simulink model "last_test"  (Simulink 7.1)
settings: Solver=ode3  StartTime=0.0  StopTime=700.0  FixedStep=0.1  RelTol=1e-3
undefined symbols (not defined in the file or in its folder): camview, kalmanfilter4
libraries: fordypningsprosjekt x7, simulink x1
settings Model: Creator=anderga  LastModifiedBy=anders
settings OptimizationCC: SimCompilerOptimization=On

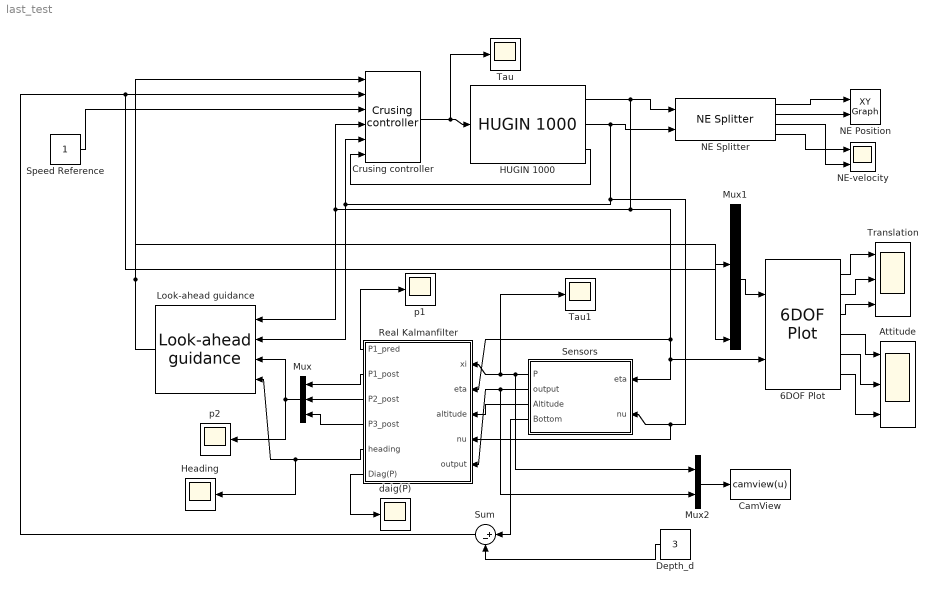
== system last_test ==
  6DOF Plot : fordypningsprosjekt/6DOF Plot  SystemSampleTime=-1
  Attitude : Scope  NumInputPorts=3
      settings: TimeRange=700  YMin=-0.5~-10~-25  YMax=0.7~1~150  SaveName=Attitude
  CamView : MATLABFcn  MATLABFcn=camview(u)
  Crusing controller : fordypningsprosjekt/Crusing controller  SystemSampleTime=-1  Kp_u=10  Ki_u=3  Kp_c=100  Kd_c=50  Kp_d=50  Kp2_d=20  Kd_d=20
  Depth_d : Constant  Orientation=left  Value=3  OutDataType=sfix(16)  OutScaling=2^0
  HUGIN 1000 : fordypningsprosjekt/HUGIN 1000  SystemSampleTime=-1  eta_0=[-30 -30 0 0 0 0]  nu_0=[0 0 0 0 0 0]  c_on_off=on  beta_c=-45  V_c=0.3
  Heading : Scope
      settings: YMin=1.3258  YMax=1.32584  SaveName=Pipeline_heading
  Look-ahead guidance : fordypningsprosjekt/Look-ahead guidance  Orientation=left  SystemSampleTime=-1
  Mux : Mux  Orientation=left  Inputs=3
  Mux1 : Mux  Inputs=6
  Mux2 : Mux  Inputs=2
  NE Position : simulink/Sinks/XY Graph  SystemSampleTime=-1  xmin=-1000  xmax=1000  ymin=-1000  ymax=1000  st=-1
  NE Splitter : fordypningsprosjekt/NE Splitter  SystemSampleTime=-1
  NE-velocity : Scope  NumInputPorts=2
      settings: YMin=1.00005~-1.87e-006  YMax=1.00011~-1.8e-006  SaveName=NE_Veloc
  Real Kalmanfilter : Subsystem  Orientation=left  AncestorBlock=fordypningsprosjekt/Real Kalmanfilter
  Sensors : Subsystem  Orientation=left  AncestorBlock=fordypningsprosjekt/Sensors
  Speed Reference : Constant  OutDataType=sfix(16)  OutScaling=2^0
  Sum : Sum  Orientation=left  Inputs=|+-  OutDataType=sfix(16)  OutScaling=2^0
  Tau : Scope
      settings: YMin=-20  YMax=110
  Tau1 : Scope
      settings: TimeRange=700  YMin=-0.5  YMax=0.5  SaveName=Cam_output
  Translation : Scope  NumInputPorts=3
      settings: YMin=-40~-50~0  YMax=30~125~10  SaveName=Translation
  daig(P) : Scope
      settings: YMin=-3.46945e-18  YMax=0.1  SaveName=diag_p_apr
  p1 : Scope
      settings: YMin=-200  YMax=600  SaveName=P_pred
  p2 : Scope
      settings: YMin=-200  YMax=600  SaveName=P_post
  wires:
  Crusing controller/1 -> HUGIN 1000/1, Tau/1
  HUGIN 1000/1 -> NE Splitter/1, Real Kalmanfilter/2(eta), Sensors/1(eta), 6DOF Plot/2, Look-ahead guidance/1, Crusing controller/4
  HUGIN 1000/2 -> NE Splitter/2, Sensors/2(nu), Real Kalmanfilter/4(nu), Look-ahead guidance/2, Crusing controller/5
  NE Splitter/1 -> NE Position/1
  NE Splitter/2 -> NE Position/2
  NE Splitter/4 -> NE-velocity/1
  NE Splitter/3 -> NE-velocity/2
  HUGIN 1000/3 -> Crusing controller/6
  Sensors/1(P) -> Real Kalmanfilter/1(xi), Tau1/1, Mux2/1
  Sensors/2(output) -> Real Kalmanfilter/5(output), Mux2/2
  Sensors/3(Altitude) -> Real Kalmanfilter/3(altitude)
  Depth_d/1 -> Sum/2
  Sensors/4(Bottom) -> Sum/1
  Sum/1 -> Mux1/3, Crusing controller/2
  Speed Reference/1 -> Crusing controller/3
  Look-ahead guidance/1 -> Mux1/6, Crusing controller/1
  Real Kalmanfilter/5(heading) -> Look-ahead guidance/4, Heading/1
  Real Kalmanfilter/2(P1_post) -> Mux/1
  Real Kalmanfilter/3(P2_post) -> Mux/2
  Real Kalmanfilter/4(P3_post) -> Mux/3
  Mux/1 -> Look-ahead guidance/3, p2/1
  6DOF Plot/1 -> Translation/1
  6DOF Plot/2 -> Translation/2
  6DOF Plot/3 -> Translation/3
  6DOF Plot/4 -> Attitude/1
  6DOF Plot/5 -> Attitude/2
  6DOF Plot/6 -> Attitude/3
  Mux1/1 -> 6DOF Plot/1
  Real Kalmanfilter/1(P1_pred) -> p1/1
  Real Kalmanfilter/6(Diag(P)) -> daig(P)/1
  Mux2/1 -> CamView/1

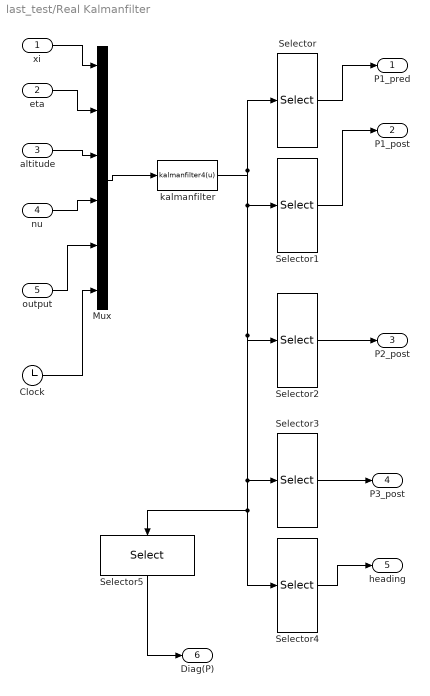
== system last_test/Real Kalmanfilter ==
  xi : Inport  OutDataType=sfix(16)  OutScaling=2^0
  eta : Inport  Port=2  OutDataType=sfix(16)  OutScaling=2^0
  altitude : Inport  Port=3  OutDataType=sfix(16)  OutScaling=2^0
  nu : Inport  Port=4  OutDataType=sfix(16)  OutScaling=2^0
  output : Inport  Port=5  OutDataType=sfix(16)  OutScaling=2^0
  Clock : Clock
      settings: Decimation=10
  Mux : Mux  Inputs=6
  Selector : Selector  InputPortWidth=17  IndexOptions=Index vector (dialog)  Indices=[1:3]  OutputSizes=1
  Selector1 : Selector  InputPortWidth=17  IndexOptions=Index vector (dialog)  Indices=4:6  OutputSizes=1
  Selector2 : Selector  InputPortWidth=17  IndexOptions=Index vector (dialog)  Indices=7:9  OutputSizes=1
  Selector3 : Selector  InputPortWidth=17  IndexOptions=Index vector (dialog)  Indices=10:12  OutputSizes=1
  Selector4 : Selector  InputPortWidth=17  IndexOptions=Index vector (dialog)  Indices=13  OutputSizes=1
  Selector5 : Selector  Orientation=down  InputPortWidth=17  IndexOptions=Index vector (dialog)  Indices=14:17  OutputSizes=1
  kalmanfilter : MATLABFcn  MATLABFcn=kalmanfilter4(u)  OutputDimensions=17
  P1_pred : Outport  OutDataType=sfix(16)  OutScaling=2^0
  P1_post : Outport  Port=2  OutDataType=sfix(16)  OutScaling=2^0
  P2_post : Outport  Port=3  OutDataType=sfix(16)  OutScaling=2^0
  P3_post : Outport  Port=4  OutDataType=sfix(16)  OutScaling=2^0
  heading : Outport  Port=5  OutDataType=sfix(16)  OutScaling=2^0
  Diag(P) : Outport  Port=6  OutDataType=sfix(16)  OutScaling=2^0
  wires:
  output/1 -> Mux/5
  Mux/1 -> kalmanfilter/1
  nu/1 -> Mux/4
  altitude/1 -> Mux/3
  eta/1 -> Mux/2
  xi/1 -> Mux/1
  kalmanfilter/1 -> Selector/1, Selector1/1, Selector2/1, Selector3/1, Selector4/1, Selector5/1
  Selector/1 -> P1_pred/1
  Selector1/1 -> P1_post/1
  Selector2/1 -> P2_post/1
  Selector3/1 -> P3_post/1
  Selector4/1 -> heading/1
  Clock/1 -> Mux/6
  Selector5/1 -> Diag(P)/1

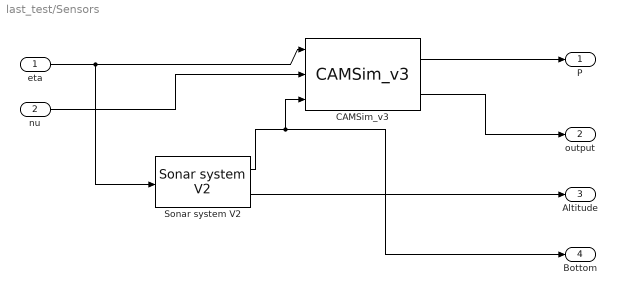
== system last_test/Sensors ==
  eta : Inport  OutDataType=sfix(16)  OutScaling=2^0
  nu : Inport  Port=2  OutDataType=sfix(16)  OutScaling=2^0
  CAMSim_v3 : fordypningsprosjekt/CAMSim_v3  SystemSampleTime=-1  noise=on  variance=0.01
      link override MATLAB Fcn: MATLABFcn=camsim3
  Sonar system V2 : fordypningsprosjekt/Sonar system V2  SystemSampleTime=-1  sea_bottom=-40
  P : Outport  OutDataType=sfix(16)  OutScaling=2^0
  output : Outport  Port=2  OutDataType=sfix(16)  OutScaling=2^0
  Altitude : Outport  Port=3  OutDataType=sfix(16)  OutScaling=2^0
  Bottom : Outport  Port=4  OutDataType=sfix(16)  OutScaling=2^0
  wires:
  eta/1 -> Sonar system V2/1, CAMSim_v3/1
  nu/1 -> CAMSim_v3/2
  Sonar system V2/1 -> Bottom/1, CAMSim_v3/3
  Sonar system V2/2 -> Altitude/1
  CAMSim_v3/1 -> P/1
  CAMSim_v3/2 -> output/1
